simulink model "Activity"  (R2024b)
settings: Solver=VariableStepAuto  StartTime=0.0  StopTime=5  RelTol=1e-3
settings Model: Creator=user  LastModifiedBy=user

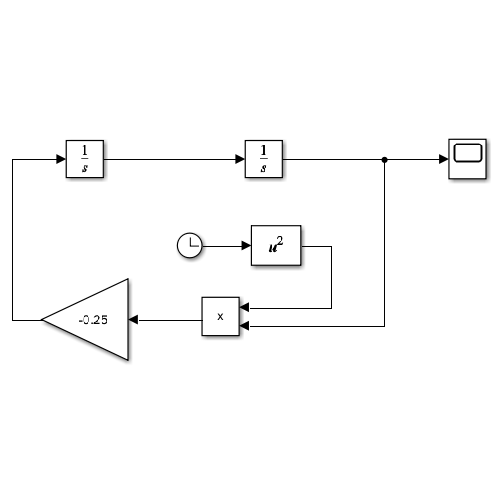
[thumbnail: Simulink's stored preview of the top-level diagram]
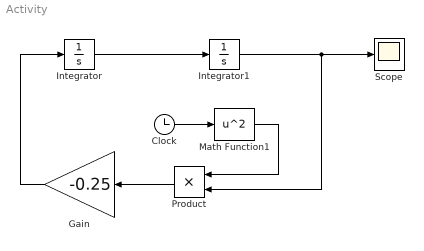
== system Activity ==
  Clock : Clock
  Gain : Gain  Gain=-0.25
  Integrator : Integrator  InitialCondition=-1
  Integrator1 : Integrator  InitialCondition=1
  Math Function1 : Math  Operator=square
  Product : Product
  Scope : Scope
  wires:
  Integrator/1 -> Integrator1/1
  Product/1 -> Gain/1
  Gain/1 -> Integrator/1
  Clock/1 -> Math Function1/1
  Math Function1/1 -> Product/1
  Integrator1/1 -> Scope/1, Product/2
